simulink model "quat_to_angles_conv"  (R2023a)
settings: Solver=VariableStepAuto  StartTime=0.0  StopTime=100  RelTol=1e-3
settings Model: Creator=ganes  LastModifiedBy=ganes

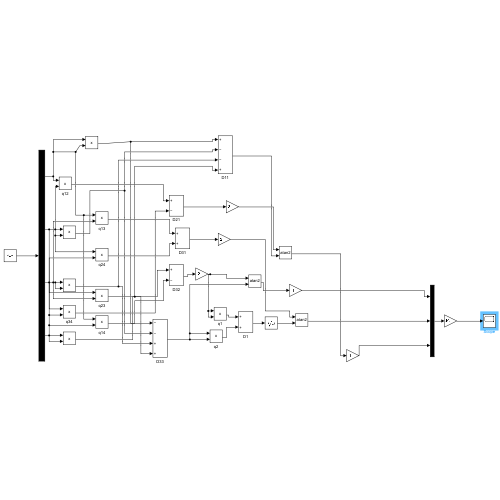
[thumbnail: Simulink's stored preview of the top-level diagram]
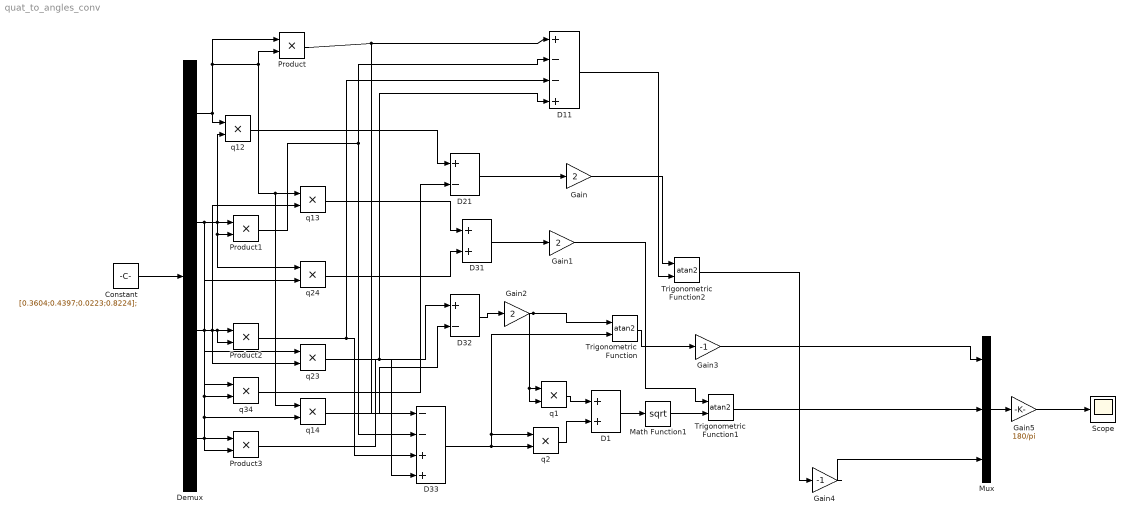
== system quat_to_angles_conv ==
  Constant : Constant  Value=[0.3604;0.4397;0.0223;0.8224];
  D1 : Sum
  D11 : Sum  Inputs=+--+
  D21 : Sum  Inputs=+-
  D31 : Sum
  D32 : Sum  Inputs=+-
  D33 : Sum  Inputs=--++
  Demux : Demux
  Gain : Gain  Gain=2
  Gain1 : Gain  Gain=2
  Gain2 : Gain  Gain=2
  Gain3 : Gain  Gain=-1
  Gain4 : Gain  Gain=-1
  Gain5 : Gain  Gain=180/pi
  Math Function1 : Math  Operator=sqrt  SignedPower=on
  Mux : Mux  Inputs=3
  Product{,1..3} (4 alike) : Product  RndMeth=Zero
  Scope : Scope
  Trigonometric Function : Trigonometry  Operator=atan2
  Trigonometric Function1 : Trigonometry  Operator=atan2
  Trigonometric Function2 : Trigonometry  Operator=atan2
  q{1..2,12..14,23..24,34} (8 alike) : Product  RndMeth=Zero
  wires:
  q13/1 -> D31/1
  Demux/4 -> q34/2, q24/2, q14/2, Product3/2, Product3/1
  q24/1 -> D31/2
  Demux/3 -> q34/1, Product2/1, Product2/2, q13/2, q23/2
  q12/1 -> D21/1
  Math Function1/1 -> Trigonometric Function1/2
  D32/1 -> Gain2/1
  D21/1 -> Gain/1
  Gain1/1 -> Trigonometric Function1/1
  Gain4/1 -> Mux/3
  D1/1 -> Math Function1/1
  Trigonometric Function1/1 -> Mux/2
  Product1/1 -> D11/2, D33/2
  Demux/2 -> q12/2, Product1/1, q24/1, Product1/2, q23/1
  q2/1 -> D1/2
  Product3/1 -> D11/4, D33/4
  D11/1 -> Trigonometric Function2/2
  Gain/1 -> Trigonometric Function2/1
  D31/1 -> Gain1/1
  Trigonometric Function/1 -> Gain3/1
  Product2/1 -> D11/3, D33/3
  Gain3/1 -> Mux/1
  Product/1 -> D11/1, D33/1
  Demux/1 -> Product/1, Product/2, q13/1, q14/1, q12/1
  q1/1 -> D1/1
  Gain2/1 -> Trigonometric Function/1, q1/2, q1/1
  q34/1 -> D21/2
  D33/1 -> Trigonometric Function/2, q2/1, q2/2
  Trigonometric Function2/1 -> Gain4/1
  q14/1 -> D32/2
  q23/1 -> D32/1
  Constant/1 -> Demux/1
  Mux/1 -> Gain5/1
  Gain5/1 -> Scope/1
